simulink model "VB_RI_EKF_GNSS_INS25"  (R2023a)
settings: Solver=FixedStepAuto  StartTime=0  StopTime=200  FixedStep=0.01  RelTol=1e-3
InitFcn:
  | %resilient_initNavigation1216;
  | %init_param;
values from neighbouring files (symbols this model uses):
  C = zeros(n,m)    [utchol.m]
undefined symbols (not defined in the file or in its folder): dt, dtDelay, g0, gam0_rad, GNSSoutragetime, ISUS_flag, magnitude, p, P0, P0_RIEKF, param, pd0, pe0, phi0_rad, pn0, psi, psi0_rad, state_dim, vd0, ve0, vn0
libraries: simulink_extras x133, simulink x81, dspstat3 x81, sharedtransform x69, sharedTrackingLibrary x17, matrix_library x15, deeplib x6, dspfactors x4, aerolibconvert2 x4, aerolibtransform2 x4, dspsrcs4 x1
(part 7 of 32)

== system VB_RI_EKF_GNSS_INS25/ISUS_RIEKF3/INS propogation ==
  note: q(1:3)
  note: Data Split
  Sensor_data : Inport
  Measuemrnt Enable Flag : Inport  Port=2
  delta_state : Inport  Port=3
  Bus Creator : BusCreator  Inputs=7
  Bus Selector : BusSelector  OutputSignals=IMU_Data.gyro_B_rad/s_LPF,IMU_Data.accl_B_m/s2_LPF,MAGN_Data,QGC_sensor_reinit,GPS_Data.pos_N_gps,GPS_Data.pos_E_gps,GPS_Data.pos_D_gps,GPS_Data.vn_gps,GPS_Data.ve_gps,GPS_Data.vd_gps,VairspeedData,elevator_aileron_rudder_deg
  Bus Selector1 : BusSelector  OutputSignals=DCM_b_n
  Bus Selector2 : BusSelector  OutputSignals=delta_state.KFState_dtheta,delta_state.KFState_dv,delta_state.KFState_dp,delta_state.KFState_dg,delta_state.KFState_da
  Data Store Read2 : DataStoreRead  DataStoreName=GPS_enable_RIEKF  IndexOptions=Index vector (dialog)  Indices=1  OutputSizes=1
  Data Type Conversion : DataTypeConversion  OutDataTypeStr=single  SaturateOnIntegerOverflow=off  RndMeth=Floor
  Gain : Gain  Gain=0.1
  Gain1 : Gain  Gain=-1
  Gain2 : Gain  Gain=0.1
  Gain4 : Gain  Commented=on  Gain=-1
  Goto15 : Goto  Commented=on  GotoTag=dtheta
  Goto16 : Goto  Commented=on  GotoTag=dv
  Goto17 : Goto  Commented=on  GotoTag=dp
  Goto18 : Goto  Commented=on  GotoTag=dda
  Goto20 : Goto  Commented=on  GotoTag=ddg
  Init_PVQ : Subsystem
  Memory : Memory
  Mux : Mux  Inputs=3
  Mux1 : Mux  Inputs=3
  Reshape : Reshape  Commented=on
  Scope : Scope
  Selector : Selector  Commented=on  InputPortWidth=15  IndexOptions=Index vector (dialog)  Indices=[1 2 3]  OutputSizes=1
  Selector1 : Selector  Commented=on  InputPortWidth=15  IndexOptions=Index vector (dialog)  Indices=[4 5 6]  OutputSizes=1
  Selector2 : Selector  Commented=on  InputPortWidth=15  IndexOptions=Index vector (dialog)  Indices=[7 8 9]  OutputSizes=1
  Selector3 : Selector  Commented=on  InputPortWidth=15  IndexOptions=Index vector (dialog)  Indices=[10 11 12]  OutputSizes=1
  Selector4 : Selector  Commented=on  InputPortWidth=15  IndexOptions=Index vector (dialog)  Indices=[13 14 15]  OutputSizes=1
  accl bias compensation : Subsystem
  att update : Subsystem
  gyro bias compensation : Subsystem
  vel/pos update : Subsystem
  INSstate : Outport
  wires:
  delta_state/1 -> Memory/1
  Gain2/1 -> accl bias compensation/3(dda)
  Gain/1 -> gyro bias compensation/2(ddg)
  Gain4/1 -> Goto15/1
  Selector/1 -> Gain4/1
  Selector1/1 -> Goto16/1
  Selector2/1 -> Goto17/1
  Reshape/1 -> Selector2/1, Selector1/1, Selector3/1, Selector/1, Selector4/1
  Selector4/1 -> Goto18/1
  Selector3/1 -> Goto20/1
  Memory/1 -> Bus Selector2/1
  [dtheta] -> att update/1(dtheta)
  [dda] -> Gain2/1
  [ddg] -> Gain/1
  Bus Selector/12 -> [elevator_aileron_rudder_deg]  "<elevator_aileron_rudder_deg>"
  Bus Creator/1 -> INSstate/1
  Bus Selector/11 -> [TAS]  "<VairspeedData>"
  Gain1/1 -> [dtheta]
  [QGC_init] -> accl bias compensation/1(QGC_init), gyro bias compensation/4(QGC_init)
  [dtheta] -> vel/pos update/1(dtheta)
  Mux/1 -> [pos_NED]
  Init_PVQ/1(quat_0) -> att update/3(quat_0)
  [accl_raw] -> vel/pos update/3(Ab)
  [QGC_init] -> att update/4(init_flag)
  Bus Selector/10 -> Mux1/3  "<vd_gps>"
  [vel_NED] -> Data Type Conversion/1
  Bus Selector/7 -> Mux/3  "<pos_D_gps>"
  Bus Selector/8 -> Mux1/1  "<vn_gps>"
  Bus Selector/5 -> Mux/1  "<pos_N_gps>"
  [gyro_raw] -> att update/2(gyro)
  Bus Selector/6 -> Mux/2  "<pos_E_gps>"
  Bus Selector/3 -> [Magn]  "<MAGN_Data>"
  Mux1/1 -> [vel_NED]
  Sensor_data/1 -> Bus Selector/1
  [fbxyz] -> Init_PVQ/2(accl_B_m/s2_LPF)
  Init_PVQ/2(v0) -> vel/pos update/4(v0)
  Init_PVQ/3(p0) -> vel/pos update/5(p0)
  Bus Selector/9 -> Mux1/2  "<ve_gps>"
  [QGC_init] -> vel/pos update/6(QGC_init)
  [pos_NED] -> Init_PVQ/4(pos_NED)
  Data Type Conversion/1 -> Init_PVQ/5(vel_NED)
  [dp] -> vel/pos update/7(dp)
  [Magn] -> Init_PVQ/3(Magn_B_guess_LPF)
  Bus Selector/4 -> [QGC_init]  "<QGC_sensor_reinit>"
  Bus Selector/1 -> [gyro_raw]  "<gyro_B_rad/s_LPF>"
  Bus Selector1/1 -> vel/pos update/2(<DCM_b_n>)  "<DCM_b_n>"
  vel/pos update/2(V) -> Bus Creator/3  "INSstate_v"
  [dv] -> vel/pos update/8(dv)
  [QGC_init] -> Init_PVQ/1(QGC_sensor_reinit)
  vel/pos update/1(p_k) -> Bus Creator/2  "INSstste_p"
  [wxyz] -> Bus Creator/4  "INSstate_w"
  [fbxyz] -> Bus Creator/5  "INSstate_fb"
  att update/1(att_update1) -> Bus Selector1/1, Bus Creator/1  "RotationData"
  accl bias compensation/1(fb) -> [fbxyz]
  accl bias compensation/2(da) -> [da]
  Measuemrnt Enable Flag/1 -> gyro bias compensation/3(Measuemrnt Enable Flag)
  gyro bias compensation/1(wb) -> [wxyz]
  gyro bias compensation/2(dg) -> [dg]
  [dg] -> Bus Creator/6  "INSstate_dg"
  [da] -> Bus Creator/7  "INSstate_da"
  Bus Selector2/3 -> [dp], Scope/1  "<KFState_dp>"
  Bus Selector2/2 -> [dv]  "<KFState_dv>"
  Bus Selector2/1 -> Gain1/1  "<KFState_dtheta>"
  Bus Selector2/5 -> [dda]  "<KFState_da>"
  Bus Selector2/4 -> [ddg]  "<KFState_dg>"
  [gyro_raw] -> gyro bias compensation/1(raw <gyro_B_rad/s_LPF>)
  [accl_raw] -> accl bias compensation/2(raw <accl_B_m/s2_LPF>)
  Bus Selector/2 -> [accl_raw]  "<accl_B_m/s2_LPF>"

== system VB_RI_EKF_GNSS_INS25/ISUS_RIEKF3/INS propogation1 ==
  note: Data Split
  note: q(1:3)
  Sensor_data : Inport
  Measuemrnt Enable Flag : Inport  Port=2
  delta_state : Inport  Port=3
  Bus Creator : BusCreator  Inputs=7
  Bus Selector : BusSelector  OutputSignals=IMU_Data.gyro_B_rad/s_LPF,IMU_Data.accl_B_m/s2_LPF,MAGN_Data,QGC_sensor_reinit,GPS_Data.pos_N_gps,GPS_Data.pos_E_gps,GPS_Data.pos_D_gps,GPS_Data.vn_gps,GPS_Data.ve_gps,GPS_Data.vd_gps,VairspeedData,elevator_aileron_rudder_deg
  Bus Selector1 : BusSelector  OutputSignals=DCM_b_n
  Bus Selector2 : BusSelector  OutputSignals=delta_state.KFState_dtheta,delta_state.KFState_dv,delta_state.KFState_dp,delta_state.KFState_dg,delta_state.KFState_da
  Data Store Read2 : DataStoreRead  DataStoreName=GPS_enable_RIEKF  IndexOptions=Index vector (dialog)  Indices=1  OutputSizes=1
  Data Type Conversion : DataTypeConversion  OutDataTypeStr=single  SaturateOnIntegerOverflow=off  RndMeth=Floor
  Gain : Gain  Gain=0.1
  Gain1 : Gain  Gain=-1
  Gain2 : Gain  Gain=0.1
  Gain4 : Gain  Commented=on  Gain=-1
  Goto15 : Goto  Commented=on  GotoTag=dtheta
  Goto16 : Goto  Commented=on  GotoTag=dv
  Goto17 : Goto  Commented=on  GotoTag=dp
  Goto18 : Goto  Commented=on  GotoTag=dda
  Goto20 : Goto  Commented=on  GotoTag=ddg
  Init_PVQ : Subsystem
  Memory : Memory
  Mux : Mux  Inputs=3
  Mux1 : Mux  Inputs=3
  Reshape : Reshape  Commented=on
  Scope : Scope
  Selector : Selector  Commented=on  InputPortWidth=15  IndexOptions=Index vector (dialog)  Indices=[1 2 3]  OutputSizes=1
  Selector1 : Selector  Commented=on  InputPortWidth=15  IndexOptions=Index vector (dialog)  Indices=[4 5 6]  OutputSizes=1
  Selector2 : Selector  Commented=on  InputPortWidth=15  IndexOptions=Index vector (dialog)  Indices=[7 8 9]  OutputSizes=1
  Selector3 : Selector  Commented=on  InputPortWidth=15  IndexOptions=Index vector (dialog)  Indices=[10 11 12]  OutputSizes=1
  Selector4 : Selector  Commented=on  InputPortWidth=15  IndexOptions=Index vector (dialog)  Indices=[13 14 15]  OutputSizes=1
  accl bias compensation : Subsystem
  att update : Subsystem
  gyro bias compensation : Subsystem
  vel/pos update : Subsystem
  INSstate : Outport
  wires:
  Bus Selector/2 -> [accl_raw]  "<accl_B_m/s2_LPF>"
  [accl_raw] -> accl bias compensation/2(raw <accl_B_m/s2_LPF>)
  [gyro_raw] -> gyro bias compensation/1(raw <gyro_B_rad/s_LPF>)
  Bus Selector2/4 -> [ddg]  "<KFState_dg>"
  Bus Selector2/5 -> [dda]  "<KFState_da>"
  Bus Selector2/1 -> Gain1/1  "<KFState_dtheta>"
  Bus Selector2/2 -> [dv]  "<KFState_dv>"
  Bus Selector2/3 -> Scope/1, [dp]  "<KFState_dp>"
  [da] -> Bus Creator/7  "INSstate_da"
  [dg] -> Bus Creator/6  "INSstate_dg"
  gyro bias compensation/2(dg) -> [dg]
  gyro bias compensation/1(wb) -> [wxyz]
  Measuemrnt Enable Flag/1 -> gyro bias compensation/3(Measuemrnt Enable Flag)
  accl bias compensation/2(da) -> [da]
  accl bias compensation/1(fb) -> [fbxyz]
  att update/1(att_update1) -> Bus Creator/1, Bus Selector1/1  "RotationData"
  [fbxyz] -> Bus Creator/5  "INSstate_fb"
  [wxyz] -> Bus Creator/4  "INSstate_w"
  vel/pos update/1(p_k) -> Bus Creator/2  "INSstste_p"
  [QGC_init] -> Init_PVQ/1(QGC_sensor_reinit)
  [dv] -> vel/pos update/8(dv)
  vel/pos update/2(V) -> Bus Creator/3  "INSstate_v"
  Bus Selector1/1 -> vel/pos update/2(<DCM_b_n>)  "<DCM_b_n>"
  Bus Selector/1 -> [gyro_raw]  "<gyro_B_rad/s_LPF>"
  Bus Selector/4 -> [QGC_init]  "<QGC_sensor_reinit>"
  [Magn] -> Init_PVQ/3(Magn_B_guess_LPF)
  [dp] -> vel/pos update/7(dp)
  Data Type Conversion/1 -> Init_PVQ/5(vel_NED)
  [pos_NED] -> Init_PVQ/4(pos_NED)
  [QGC_init] -> vel/pos update/6(QGC_init)
  Bus Selector/9 -> Mux1/2  "<ve_gps>"
  Init_PVQ/3(p0) -> vel/pos update/5(p0)
  Init_PVQ/2(v0) -> vel/pos update/4(v0)
  [fbxyz] -> Init_PVQ/2(accl_B_m/s2_LPF)
  Sensor_data/1 -> Bus Selector/1
  Mux1/1 -> [vel_NED]
  Bus Selector/3 -> [Magn]  "<MAGN_Data>"
  Bus Selector/6 -> Mux/2  "<pos_E_gps>"
  [gyro_raw] -> att update/2(gyro)
  Bus Selector/5 -> Mux/1  "<pos_N_gps>"
  Bus Selector/8 -> Mux1/1  "<vn_gps>"
  Bus Selector/7 -> Mux/3  "<pos_D_gps>"
  [vel_NED] -> Data Type Conversion/1
  Bus Selector/10 -> Mux1/3  "<vd_gps>"
  [QGC_init] -> att update/4(init_flag)
  [accl_raw] -> vel/pos update/3(Ab)
  Init_PVQ/1(quat_0) -> att update/3(quat_0)
  Mux/1 -> [pos_NED]
  [dtheta] -> vel/pos update/1(dtheta)
  [QGC_init] -> gyro bias compensation/4(QGC_init), accl bias compensation/1(QGC_init)
  Gain1/1 -> [dtheta]
  Bus Selector/11 -> [TAS]  "<VairspeedData>"
  Bus Creator/1 -> INSstate/1
  Bus Selector/12 -> [elevator_aileron_rudder_deg]  "<elevator_aileron_rudder_deg>"
  [ddg] -> Gain/1
  [dda] -> Gain2/1
  [dtheta] -> att update/1(dtheta)
  Memory/1 -> Bus Selector2/1
  Selector3/1 -> Goto20/1
  Selector4/1 -> Goto18/1
  Reshape/1 -> Selector4/1, Selector/1, Selector3/1, Selector1/1, Selector2/1
  Selector2/1 -> Goto17/1
  Selector1/1 -> Goto16/1
  Selector/1 -> Gain4/1
  Gain4/1 -> Goto15/1
  Gain/1 -> gyro bias compensation/2(ddg)
  Gain2/1 -> accl bias compensation/3(dda)
  delta_state/1 -> Memory/1

== system VB_RI_EKF_GNSS_INS25/ISUS_RIEKF3/INS propogation2 ==
  note: q(1:3)
  note: Data Split
  Sensor_data : Inport
  Measuemrnt Enable Flag : Inport  Port=2
  delta_state : Inport  Port=3
  Bus Creator : BusCreator  Inputs=7
  Bus Selector : BusSelector  OutputSignals=IMU_Data.gyro_B_rad/s_LPF,IMU_Data.accl_B_m/s2_LPF,MAGN_Data,QGC_sensor_reinit,GPS_Data.pos_N_gps,GPS_Data.pos_E_gps,GPS_Data.pos_D_gps,GPS_Data.vn_gps,GPS_Data.ve_gps,GPS_Data.vd_gps,VairspeedData,elevator_aileron_rudder_deg
  Bus Selector1 : BusSelector  OutputSignals=DCM_b_n
  Bus Selector2 : BusSelector  OutputSignals=delta_state.KFState_dtheta,delta_state.KFState_dv,delta_state.KFState_dp,delta_state.KFState_dg,delta_state.KFState_da
  Data Store Read2 : DataStoreRead  DataStoreName=GPS_enable_RIEKF  IndexOptions=Index vector (dialog)  Indices=1  OutputSizes=1
  Data Type Conversion : DataTypeConversion  OutDataTypeStr=single  SaturateOnIntegerOverflow=off  RndMeth=Floor
  Gain : Gain  Gain=0.1
  Gain1 : Gain  Gain=-1
  Gain2 : Gain  Gain=0.1
  Gain4 : Gain  Commented=on  Gain=-1
  Goto15 : Goto  Commented=on  GotoTag=dtheta
  Goto16 : Goto  Commented=on  GotoTag=dv
  Goto17 : Goto  Commented=on  GotoTag=dp
  Goto18 : Goto  Commented=on  GotoTag=dda
  Goto20 : Goto  Commented=on  GotoTag=ddg
  Init_PVQ : Subsystem
  Memory : Memory
  Mux : Mux  Inputs=3
  Mux1 : Mux  Inputs=3
  Reshape : Reshape  Commented=on
  Scope : Scope
  Selector : Selector  Commented=on  InputPortWidth=15  IndexOptions=Index vector (dialog)  Indices=[1 2 3]  OutputSizes=1
  Selector1 : Selector  Commented=on  InputPortWidth=15  IndexOptions=Index vector (dialog)  Indices=[4 5 6]  OutputSizes=1
  Selector2 : Selector  Commented=on  InputPortWidth=15  IndexOptions=Index vector (dialog)  Indices=[7 8 9]  OutputSizes=1
  Selector3 : Selector  Commented=on  InputPortWidth=15  IndexOptions=Index vector (dialog)  Indices=[10 11 12]  OutputSizes=1
  Selector4 : Selector  Commented=on  InputPortWidth=15  IndexOptions=Index vector (dialog)  Indices=[13 14 15]  OutputSizes=1
  accl bias compensation : Subsystem
  att update : Subsystem
  gyro bias compensation : Subsystem
  vel/pos update : Subsystem
  INSstate : Outport
  wires:
  delta_state/1 -> Memory/1
  Gain2/1 -> accl bias compensation/3(dda)
  Gain/1 -> gyro bias compensation/2(ddg)
  Gain4/1 -> Goto15/1
  Selector/1 -> Gain4/1
  Selector1/1 -> Goto16/1
  Selector2/1 -> Goto17/1
  Reshape/1 -> Selector2/1, Selector1/1, Selector3/1, Selector/1, Selector4/1
  Selector4/1 -> Goto18/1
  Selector3/1 -> Goto20/1
  Memory/1 -> Bus Selector2/1
  [dtheta] -> att update/1(dtheta)
  [dda] -> Gain2/1
  [ddg] -> Gain/1
  Bus Selector/12 -> [elevator_aileron_rudder_deg]  "<elevator_aileron_rudder_deg>"
  Bus Creator/1 -> INSstate/1
  Bus Selector/11 -> [TAS]  "<VairspeedData>"
  Gain1/1 -> [dtheta]
  [QGC_init] -> accl bias compensation/1(QGC_init), gyro bias compensation/4(QGC_init)
  [dtheta] -> vel/pos update/1(dtheta)
  Mux/1 -> [pos_NED]
  Init_PVQ/1(quat_0) -> att update/3(quat_0)
  [accl_raw] -> vel/pos update/3(Ab)
  [QGC_init] -> att update/4(init_flag)
  Bus Selector/10 -> Mux1/3  "<vd_gps>"
  [vel_NED] -> Data Type Conversion/1
  Bus Selector/7 -> Mux/3  "<pos_D_gps>"
  Bus Selector/8 -> Mux1/1  "<vn_gps>"
  Bus Selector/5 -> Mux/1  "<pos_N_gps>"
  [gyro_raw] -> att update/2(gyro)
  Bus Selector/6 -> Mux/2  "<pos_E_gps>"
  Bus Selector/3 -> [Magn]  "<MAGN_Data>"
  Mux1/1 -> [vel_NED]
  Sensor_data/1 -> Bus Selector/1
  [fbxyz] -> Init_PVQ/2(accl_B_m/s2_LPF)
  Init_PVQ/2(v0) -> vel/pos update/4(v0)
  Init_PVQ/3(p0) -> vel/pos update/5(p0)
  Bus Selector/9 -> Mux1/2  "<ve_gps>"
  [QGC_init] -> vel/pos update/6(QGC_init)
  [pos_NED] -> Init_PVQ/4(pos_NED)
  Data Type Conversion/1 -> Init_PVQ/5(vel_NED)
  [dp] -> vel/pos update/7(dp)
  [Magn] -> Init_PVQ/3(Magn_B_guess_LPF)
  Bus Selector/4 -> [QGC_init]  "<QGC_sensor_reinit>"
  Bus Selector/1 -> [gyro_raw]  "<gyro_B_rad/s_LPF>"
  Bus Selector1/1 -> vel/pos update/2(<DCM_b_n>)  "<DCM_b_n>"
  vel/pos update/2(V) -> Bus Creator/3  "INSstate_v"
  [dv] -> vel/pos update/8(dv)
  [QGC_init] -> Init_PVQ/1(QGC_sensor_reinit)
  vel/pos update/1(p_k) -> Bus Creator/2  "INSstste_p"
  [wxyz] -> Bus Creator/4  "INSstate_w"
  [fbxyz] -> Bus Creator/5  "INSstate_fb"
  att update/1(att_update1) -> Bus Selector1/1, Bus Creator/1  "RotationData"
  accl bias compensation/1(fb) -> [fbxyz]
  accl bias compensation/2(da) -> [da]
  Measuemrnt Enable Flag/1 -> gyro bias compensation/3(Measuemrnt Enable Flag)
  gyro bias compensation/1(wb) -> [wxyz]
  gyro bias compensation/2(dg) -> [dg]
  [dg] -> Bus Creator/6  "INSstate_dg"
  [da] -> Bus Creator/7  "INSstate_da"
  Bus Selector2/3 -> [dp], Scope/1  "<KFState_dp>"
  Bus Selector2/2 -> [dv]  "<KFState_dv>"
  Bus Selector2/1 -> Gain1/1  "<KFState_dtheta>"
  Bus Selector2/5 -> [dda]  "<KFState_da>"
  Bus Selector2/4 -> [ddg]  "<KFState_dg>"
  [gyro_raw] -> gyro bias compensation/1(raw <gyro_B_rad/s_LPF>)
  [accl_raw] -> accl bias compensation/2(raw <accl_B_m/s2_LPF>)
  Bus Selector/2 -> [accl_raw]  "<accl_B_m/s2_LPF>"

== system VB_RI_EKF_GNSS_INS25/ISUS_RIEKF3/INS propogation3 ==
  note: Data Split
  note: q(1:3)
  Sensor_data : Inport
  Measuemrnt Enable Flag : Inport  Port=2
  delta_state : Inport  Port=3
  Bus Creator : BusCreator  Inputs=7
  Bus Selector : BusSelector  OutputSignals=IMU_Data.gyro_B_rad/s_LPF,IMU_Data.accl_B_m/s2_LPF,MAGN_Data,QGC_sensor_reinit,GPS_Data.pos_N_gps,GPS_Data.pos_E_gps,GPS_Data.pos_D_gps,GPS_Data.vn_gps,GPS_Data.ve_gps,GPS_Data.vd_gps,VairspeedData,elevator_aileron_rudder_deg
  Bus Selector1 : BusSelector  OutputSignals=DCM_b_n
  Bus Selector2 : BusSelector  OutputSignals=delta_state.KFState_dtheta,delta_state.KFState_dv,delta_state.KFState_dp,delta_state.KFState_dg,delta_state.KFState_da
  Data Store Read2 : DataStoreRead  DataStoreName=GPS_enable_RIEKF  IndexOptions=Index vector (dialog)  Indices=1  OutputSizes=1
  Data Type Conversion : DataTypeConversion  OutDataTypeStr=single  SaturateOnIntegerOverflow=off  RndMeth=Floor
  Gain : Gain  Gain=0.1
  Gain1 : Gain  Gain=-1
  Gain2 : Gain  Gain=0.1
  Gain4 : Gain  Commented=on  Gain=-1
  Goto15 : Goto  Commented=on  GotoTag=dtheta
  Goto16 : Goto  Commented=on  GotoTag=dv
  Goto17 : Goto  Commented=on  GotoTag=dp
  Goto18 : Goto  Commented=on  GotoTag=dda
  Goto20 : Goto  Commented=on  GotoTag=ddg
  Init_PVQ : Subsystem
  Memory : Memory
  Mux : Mux  Inputs=3
  Mux1 : Mux  Inputs=3
  Reshape : Reshape  Commented=on
  Scope : Scope
  Selector : Selector  Commented=on  InputPortWidth=15  IndexOptions=Index vector (dialog)  Indices=[1 2 3]  OutputSizes=1
  Selector1 : Selector  Commented=on  InputPortWidth=15  IndexOptions=Index vector (dialog)  Indices=[4 5 6]  OutputSizes=1
  Selector2 : Selector  Commented=on  InputPortWidth=15  IndexOptions=Index vector (dialog)  Indices=[7 8 9]  OutputSizes=1
  Selector3 : Selector  Commented=on  InputPortWidth=15  IndexOptions=Index vector (dialog)  Indices=[10 11 12]  OutputSizes=1
  Selector4 : Selector  Commented=on  InputPortWidth=15  IndexOptions=Index vector (dialog)  Indices=[13 14 15]  OutputSizes=1
  accl bias compensation : Subsystem
  att update : Subsystem
  gyro bias compensation : Subsystem
  vel/pos update : Subsystem
  INSstate : Outport
  wires:
  Bus Selector/2 -> [accl_raw]  "<accl_B_m/s2_LPF>"
  [accl_raw] -> accl bias compensation/2(raw <accl_B_m/s2_LPF>)
  [gyro_raw] -> gyro bias compensation/1(raw <gyro_B_rad/s_LPF>)
  Bus Selector2/4 -> [ddg]  "<KFState_dg>"
  Bus Selector2/5 -> [dda]  "<KFState_da>"
  Bus Selector2/1 -> Gain1/1  "<KFState_dtheta>"
  Bus Selector2/2 -> [dv]  "<KFState_dv>"
  Bus Selector2/3 -> Scope/1, [dp]  "<KFState_dp>"
  [da] -> Bus Creator/7  "INSstate_da"
  [dg] -> Bus Creator/6  "INSstate_dg"
  gyro bias compensation/2(dg) -> [dg]
  gyro bias compensation/1(wb) -> [wxyz]
  Measuemrnt Enable Flag/1 -> gyro bias compensation/3(Measuemrnt Enable Flag)
  accl bias compensation/2(da) -> [da]
  accl bias compensation/1(fb) -> [fbxyz]
  att update/1(att_update1) -> Bus Creator/1, Bus Selector1/1  "RotationData"
  [fbxyz] -> Bus Creator/5  "INSstate_fb"
  [wxyz] -> Bus Creator/4  "INSstate_w"
  vel/pos update/1(p_k) -> Bus Creator/2  "INSstste_p"
  [QGC_init] -> Init_PVQ/1(QGC_sensor_reinit)
  [dv] -> vel/pos update/8(dv)
  vel/pos update/2(V) -> Bus Creator/3  "INSstate_v"
  Bus Selector1/1 -> vel/pos update/2(<DCM_b_n>)  "<DCM_b_n>"
  Bus Selector/1 -> [gyro_raw]  "<gyro_B_rad/s_LPF>"
  Bus Selector/4 -> [QGC_init]  "<QGC_sensor_reinit>"
  [Magn] -> Init_PVQ/3(Magn_B_guess_LPF)
  [dp] -> vel/pos update/7(dp)
  Data Type Conversion/1 -> Init_PVQ/5(vel_NED)
  [pos_NED] -> Init_PVQ/4(pos_NED)
  [QGC_init] -> vel/pos update/6(QGC_init)
  Bus Selector/9 -> Mux1/2  "<ve_gps>"
  Init_PVQ/3(p0) -> vel/pos update/5(p0)
  Init_PVQ/2(v0) -> vel/pos update/4(v0)
  [fbxyz] -> Init_PVQ/2(accl_B_m/s2_LPF)
  Sensor_data/1 -> Bus Selector/1
  Mux1/1 -> [vel_NED]
  Bus Selector/3 -> [Magn]  "<MAGN_Data>"
  Bus Selector/6 -> Mux/2  "<pos_E_gps>"
  [gyro_raw] -> att update/2(gyro)
  Bus Selector/5 -> Mux/1  "<pos_N_gps>"
  Bus Selector/8 -> Mux1/1  "<vn_gps>"
  Bus Selector/7 -> Mux/3  "<pos_D_gps>"
  [vel_NED] -> Data Type Conversion/1
  Bus Selector/10 -> Mux1/3  "<vd_gps>"
  [QGC_init] -> att update/4(init_flag)
  [accl_raw] -> vel/pos update/3(Ab)
  Init_PVQ/1(quat_0) -> att update/3(quat_0)
  Mux/1 -> [pos_NED]
  [dtheta] -> vel/pos update/1(dtheta)
  [QGC_init] -> gyro bias compensation/4(QGC_init), accl bias compensation/1(QGC_init)
  Gain1/1 -> [dtheta]
  Bus Selector/11 -> [TAS]  "<VairspeedData>"
  Bus Creator/1 -> INSstate/1
  Bus Selector/12 -> [elevator_aileron_rudder_deg]  "<elevator_aileron_rudder_deg>"
  [ddg] -> Gain/1
  [dda] -> Gain2/1
  [dtheta] -> att update/1(dtheta)
  Memory/1 -> Bus Selector2/1
  Selector3/1 -> Goto20/1
  Selector4/1 -> Goto18/1
  Reshape/1 -> Selector4/1, Selector/1, Selector3/1, Selector1/1, Selector2/1
  Selector2/1 -> Goto17/1
  Selector1/1 -> Goto16/1
  Selector/1 -> Gain4/1
  Gain4/1 -> Goto15/1
  Gain/1 -> gyro bias compensation/2(ddg)
  Gain2/1 -> accl bias compensation/3(dda)
  delta_state/1 -> Memory/1

== system VB_RI_EKF_GNSS_INS25/ISUS_RIEKF3/Subsystem ==
  EKFstate_M1 : Inport
  EKFstate_M2 : Inport  Port=2
  EKFstate_M3 : Inport  Port=3
  Bus Selector : BusSelector  OutputSignals=delta_state,covariance,beta1
  Bus Selector1 : BusSelector  OutputSignals=delta_state,covariance,m_innov_z0,Sk_z0,beta2
  Bus Selector2 : BusSelector  OutputSignals=delta_state,covariance,m_innov_z0,Sk_z0,beta3
  Constant1 : Constant  Value=P0_RIEKF  OutDataTypeStr=single
  Constant6 : Constant  Value=zeros(15,1)  OutDataTypeStr=single
  Constant7 : Constant  Value=P0_RIEKF  OutDataTypeStr=single
  Delay{,1..3,5..7} (7 alike) : Delay  DelayLength=1  InitialConditionSource=Input port
      settings: InputPortMap=u0,p4
  Display : Display
  Display1 : Display
  Display2 : Display
  Gain : Gain  Gain=3
  ISIU : Subsystem
  Reshape2 : Reshape  OutputDimensionality=Column vector (2-D)
  Subsystem : Subsystem
  Subsystem1 : Subsystem
  Subsystem2 : Subsystem
  Subsystem3 : Subsystem
  P_mixed_RIEKF_M1 : Outport
  X_mixed_RIEKF_M1 : Outport  Port=2
  P_mixed_RIEKF_M2 : Outport  Port=3
  X_mixed_RIEKF_M2 : Outport  Port=4
  xk_k : Outport  Port=5
  pk_k : Outport  Port=6
  X_mixed_RIEKF_M3 : Outport  Port=7
  P_mixed_RIEKF_M3 : Outport  Port=8
  beta_1 : Outport  Port=9
  beta_2 : Outport  Port=10
  beta_3 : Outport  Port=11
  wires:
  Bus Selector2/1 -> ISIU/3(xk_k_3)  "<delta_state>"
  EKFstate_M3/1 -> Bus Selector2/1
  ISIU/8(pk_k_o3) -> Delay7/1
  Delay7/1 -> P_mixed_RIEKF_M3/1
  ISIU/5(xk_k_o3) -> Delay6/1
  Reshape2/1 -> Delay/2, Delay3/2, Delay6/2
  Delay6/1 -> Subsystem3/1(X_mixed_RIEKF_M1)
  ISIU/1(xk_k) -> Subsystem/1(X_mixed_RIEKF_M1)
  Subsystem/1(Out1) -> xk_k/1  "xk_k"
  Constant1/1 -> Delay5/2
  ISIU/2(pk_k) -> Delay5/1
  Delay5/1 -> pk_k/1
  Delay3/1 -> Subsystem2/1(X_mixed_RIEKF_M1)
  Delay1/1 -> P_mixed_RIEKF_M1/1
  ISIU/3(xk_k_o1) -> Delay/1  "X_mixed_RIEKF_M1"
  EKFstate_M1/1 -> Bus Selector/1
  ISIU/6(pk_k_o1) -> Delay1/1
  Bus Selector/1 -> ISIU/1(xk_k_1)  "<delta_state>"
  Delay2/1 -> P_mixed_RIEKF_M2/1
  Constant6/1 -> Reshape2/1
  ISIU/7(pk_k_o2) -> Delay2/1
  ISIU/4(xk_k_o2) -> Delay3/1  "X_mixed_RIEKF_M2"
  EKFstate_M2/1 -> Bus Selector1/1
  Delay/1 -> Subsystem1/1(X_mixed_RIEKF_M1)
  Bus Selector1/1 -> ISIU/2(xk_k_2)  "<delta_state>"
  Constant7/1 -> Gain/1
  Bus Selector/2 -> ISIU/4(pk_k_1)  "<covariance>"
  Bus Selector1/2 -> ISIU/5(pk_k_2)  "<covariance>"
  Bus Selector2/2 -> ISIU/6(pk_k_3)  "<covariance>"
  Subsystem1/1(Out1) -> X_mixed_RIEKF_M1/1  "xk_k"
  Subsystem2/1(Out1) -> X_mixed_RIEKF_M2/1  "xk_k"
  Subsystem3/1(Out1) -> X_mixed_RIEKF_M3/1  "xk_k"
  Gain/1 -> Delay1/2, Delay2/2, Delay7/2
  Bus Selector/3 -> ISIU/7(beta1)  "<beta1>"
  Bus Selector1/5 -> ISIU/8(beta2)  "<beta2>"
  Bus Selector2/5 -> ISIU/9(beta3)  "<beta3>"
  ISIU/9(beta_1) -> Display/1, beta_1/1
  ISIU/10(beta_2) -> Display1/1, beta_2/1
  ISIU/11(beta_3) -> Display2/1, beta_3/1

== system VB_RI_EKF_GNSS_INS25/No.1_Sensor_Data_Process/GPS_Data_Process ==
  note: GPS_fixtype:
      | 0: 定位不可用或无效
      | 1:单点定位
      | 2:伪距差分
      | 4:RTK固定解
  GPS_Vecef_m/s : Inport
  GPS_LLA_rad : Inport  Port=2
  GPS_fixtype : Inport  Port=3
  hdop_GPS : Inport  Port=4
  QGC_sensor_reinit : Inport  Port=5
  Bus Creator : BusCreator  Inputs=13
  Demux : Demux  Outputs=3
  Demux1 : Demux  Outputs=3
  Demux3 : Demux  Outputs=3
  GPS_fixtype1 : InportShadow  Port=3
  LLA2NED : Subsystem
  heading_GPS : Subsystem
  GPS_Data : Outport
  GPS0 : Outport  Port=2
  GPS_noerr : Outport  Port=3
  wires:
  hdop_GPS/1 -> Bus Creator/13  "hdop_GPS"
  heading_GPS/2(heading_GPS_valid) -> Bus Creator/11  "heading_GPS_valid"
  heading_GPS/1(heading_GPS_rad) -> Bus Creator/10  "heading_GPS_rad"
  LLA2NED/2(gpsvNEDout) -> heading_GPS/1(Vned), Demux/1
  GPS_Vecef_m/s/1 -> LLA2NED/3(GPS_Vecef_m/s)
  Demux1/3 -> Bus Creator/6  "pos_D_gps"
  Demux1/2 -> Bus Creator/5  "pos_E_gps"
  Demux1/1 -> Bus Creator/4  "pos_N_gps"
  QGC_sensor_reinit/1 -> LLA2NED/4(QGC_sensor_reinit)  "QGC_sensor_reinit"
  GPS_fixtype/1 -> Bus Creator/12  "fixtype_gps"
  Demux3/1 -> Bus Creator/1  "lat_gps"
  Demux3/2 -> Bus Creator/2  "lon_gps"
  Demux/2 -> Bus Creator/8  "ve_gps"
  GPS_LLA_rad/1 -> LLA2NED/1(gps_LLA_rad), Demux3/1
  Demux/1 -> Bus Creator/7  "vn_gps"
  Demux/3 -> Bus Creator/9  "vd_gps"
  Demux3/3 -> Bus Creator/3  "H_gps"
  Bus Creator/1 -> GPS_Data/1
  GPS_fixtype1/1 -> LLA2NED/2(GPSfixtype)  "fixtype_gps"
  LLA2NED/1("gpsposNEDout ") -> Demux1/1
  LLA2NED/3(GPS0) -> GPS0/1
  LLA2NED/4(gpsposNED_noerr) -> GPS_noerr/1

== system VB_RI_EKF_GNSS_INS25/No.1_Sensor_Data_Process/IMU_Data_Process ==
  gyro_B_rad/s_ori : Inport
  accl_B_m/s_ori : Inport  Port=2
  Bias Eliminate : Subsystem
  Bus Creator : BusCreator  Inputs=2
  accl_preprocessing2 : Subsystem  Commented=on
  gyro_preprocessing2 : Subsystem  Commented=on
  IMU_Data : Outport  PortDimensions=6
  wires:
  gyro_B_rad/s_ori/1 -> Bias Eliminate/1(gyro_B_rad/s_ori)  "gyro_B_rad/s_LPF"
  Bias Eliminate/1(Out1) -> Bus Creator/1  "gyro_B_rad/s_LPF"
  accl_B_m/s_ori/1 -> Bus Creator/2  "accl_B_m/s2_LPF"
  Bus Creator/1 -> IMU_Data/1

== system VB_RI_EKF_GNSS_INS25/No.1_Sensor_Data_Process/Magn_Data_Process ==
  magn_B_guass_ori : Inport
  Data Type Conversion : DataTypeConversion  OutDataTypeStr=single  SaturateOnIntegerOverflow=off  RndMeth=Floor
  MATLAB Function1 : MATLAB Function  Commented=on  TreatAsAtomicUnit=on
  Magn_preprocessing : Subsystem
  MAGN_Data : Outport
  wires:
  magn_B_guass_ori/1 -> Data Type Conversion/1, Magn_preprocessing/1(Magn_B_rad/s_ori)
  Data Type Conversion/1 -> MAGN_Data/1

== system VB_RI_EKF_GNSS_INS25/No.1_Sensor_Data_Process/Subsystem ==
  Vairspeed : Inport
  Constant : Constant  Value=0  OutDataTypeStr=single
  Mux : Mux  Inputs=3
  TD_baro : Subsystem
  Terminator : Terminator
  VairspeedData : Outport
  wires:
  TD_baro/2(H_baro_TD) -> Mux/1
  Constant/1 -> Mux/3, Mux/2
  Mux/1 -> VairspeedData/1  "VairspeedData"
  Vairspeed/1 -> TD_baro/1(H_baro)
  TD_baro/1(vH_baro_TD) -> Terminator/1  "vH_baro_m/s_TD"

== system VB_RI_EKF_GNSS_INS25/No.1_Sensor_Data_Process/TOF_Data_Process ==
  TOF_mm_ori : Inport
  QGC_sensor_reinit : Inport  Port=2
  Bus Creator1 : BusCreator  Inputs=4
  Data Type Conversion : DataTypeConversion  OutDataTypeStr=uint8  SaturateOnIntegerOverflow=off  RndMeth=Floor
  Data Type Conversion1 : DataTypeConversion  OutDataTypeStr=single  SaturateOnIntegerOverflow=off  RndMeth=Floor
  Demux : Demux  Outputs=3
  Gain : Gain  Gain=0.01
  Scope : Scope  NumInputPorts=2
  Scope1 : Scope  NumInputPorts=2
  Sum : Sum  Inputs=|-+
  TD_baro : Subsystem
  reinit_TOF : Subsystem
  TOF_Data : Outport
  wires:
  Sum/1 -> Data Type Conversion1/1, Scope1/2  "TOF_Dist_m"
  reinit_TOF/1(dataout) -> Sum/1, Scope1/1
  QGC_sensor_reinit/1 -> reinit_TOF/1(QGC_sensor_reinit)
  Data Type Conversion/1 -> Bus Creator1/4  "TOF_sts"
  Gain/1 -> reinit_TOF/2(Data), Sum/2  "TOF_Dist_m"
  TD_baro/1(vH_TOF_TD) -> Bus Creator1/1, Scope/1  "vH_TOF_m/s_TD"
  Bus Creator1/1 -> TOF_Data/1  "TOF_Data"
  Demux/2 -> Bus Creator1/3  "TOF_Inten"
  TOF_mm_ori/1 -> Demux/1
  Demux/1 -> Gain/1
  Demux/3 -> Data Type Conversion/1  "TOF_sts"
  TD_baro/2(H_TOF_TD) -> Scope/2, Bus Creator1/2  "H_TOF_TD"
  Data Type Conversion1/1 -> TD_baro/1(H_TOF)  "补偿姿态前"

== system VB_RI_EKF_GNSS_INS25/No.1_Sensor_Data_Process/baro_Data_Process ==
  baro : Inport
  QGC_sensor_reinit : Inport  Port=2
  baro_tem : Inport  Port=3
  Bus Creator : BusCreator  Inputs=2
  Constant : Constant  Value=0  OutDataTypeStr=single
  From Workspace : FromWorkspace  Commented=on  VariableName=[All.t',All.Alt_Ps]
  Gain : Gain  Gain=0.01
  Pressure2Height : Subsystem
  Scope : Scope
  Scope1 : Scope  Commented=on  NumInputPorts=2
  Sum : Sum  Inputs=|+-
  Sum1 : Sum  Commented=on  Inputs=|+-
  Sum2 : Sum  Inputs=|+-
  Switch : Switch  Criteria=u2 > Threshold  Threshold=31  SaturateOnIntegerOverflow=off  InputSameDT=off
  TD_baro : Subsystem
  TemCompensate1 : Subsystem
  reinit_baro0 : Subsystem
  reinit_baro1 : Subsystem  Commented=on
  BARO_Data : Outport  PortDimensions=2
  wires:
  baro_tem/1 -> TemCompensate1/1(baro_tem), Switch/2  "AFCbarotem"
  Pressure2Height/1(H_baro) -> TD_baro/1(H_baro)  "AFC4"
  Switch/1 -> Sum2/2
  baro/1 -> Gain/1  "AFC4"
  Constant/1 -> Switch/1
  TemCompensate1/1(bias) -> Switch/3
  Sum2/1 -> Sum/1, reinit_baro0/2(Data)
  TD_baro/2(H_baro_TD) -> Sum2/1  "H_baro_TD"
  Sum/1 -> Scope1/2, Scope/1, Bus Creator/2  "H_baro_TD"
  reinit_baro0/1(dataout) -> Sum/2
  QGC_sensor_reinit/1 -> reinit_baro1/1(QGC_sensor_reinit), reinit_baro0/1(QGC_sensor_reinit)
  Bus Creator/1 -> BARO_Data/1
  Gain/1 -> Pressure2Height/1(baro)
  TD_baro/1(vH_baro_TD) -> Bus Creator/1  "vH_baro_m/s_TD"
  From Workspace/1 -> reinit_baro1/2(Data), Sum1/1
  reinit_baro1/1(dataout) -> Sum1/2
  Sum1/1 -> Scope1/1

== system VB_RI_EKF_GNSS_INS25/No.1_Sensor_Data_Process1/GPS_Data_Process ==
  note: GPS_fixtype:
      | 0: 定位不可用或无效
      | 1:单点定位
      | 2:伪距差分
      | 4:RTK固定解
  GPS_Vecef_m/s : Inport
  GPS_LLA_rad : Inport  Port=2
  GPS_fixtype : Inport  Port=3
  hdop_GPS : Inport  Port=4
  QGC_sensor_reinit : Inport  Port=5
  GPS0 : Inport  Port=6
  Bus Creator : BusCreator  Inputs=13
  Demux : Demux  Outputs=3
  Demux1 : Demux  Outputs=3
  Demux3 : Demux  Outputs=3
  GPS_fixtype1 : InportShadow  Port=3
  LLA2NED : Subsystem
  heading_GPS : Subsystem
  GPS_Data : Outport
  wires:
  LLA2NED/1("gpsposNEDout ") -> Demux1/1
  GPS_fixtype1/1 -> LLA2NED/2(GPSfixtype)  "fixtype_gps"
  Bus Creator/1 -> GPS_Data/1
  Demux3/3 -> Bus Creator/3  "H_gps"
  Demux/3 -> Bus Creator/9  "vd_gps"
  Demux/1 -> Bus Creator/7  "vn_gps"
  GPS_LLA_rad/1 -> Demux3/1, LLA2NED/1(gps_LLA_rad)
  Demux/2 -> Bus Creator/8  "ve_gps"
  Demux3/2 -> Bus Creator/2  "lon_gps"
  Demux3/1 -> Bus Creator/1  "lat_gps"
  GPS_fixtype/1 -> Bus Creator/12  "fixtype_gps"
  QGC_sensor_reinit/1 -> LLA2NED/4(QGC_sensor_reinit)  "QGC_sensor_reinit"
  Demux1/1 -> Bus Creator/4  "pos_N_gps"
  Demux1/2 -> Bus Creator/5  "pos_E_gps"
  Demux1/3 -> Bus Creator/6  "pos_D_gps"
  GPS_Vecef_m/s/1 -> LLA2NED/3(GPS_Vecef_m/s)
  LLA2NED/2(gpsvNEDout) -> Demux/1, heading_GPS/1(Vned)
  heading_GPS/1(heading_GPS_rad) -> Bus Creator/10  "heading_GPS_rad"
  heading_GPS/2(heading_GPS_valid) -> Bus Creator/11  "heading_GPS_valid"
  hdop_GPS/1 -> Bus Creator/13  "hdop_GPS"
  GPS0/1 -> LLA2NED/5(GPS0)

== system VB_RI_EKF_GNSS_INS25/No.1_Sensor_Data_Process1/IMU_Data_Process ==
  gyro_B_rad/s_ori : Inport
  accl_B_m/s_ori : Inport  Port=2
  Bias Eliminate : Subsystem
  Bus Creator : BusCreator  Inputs=2
  accl_preprocessing2 : Subsystem  Commented=on
  gyro_preprocessing2 : Subsystem  Commented=on
  IMU_Data : Outport  PortDimensions=6
  wires:
  Bus Creator/1 -> IMU_Data/1
  accl_B_m/s_ori/1 -> Bus Creator/2  "accl_B_m/s2_LPF"
  Bias Eliminate/1(Out1) -> Bus Creator/1  "gyro_B_rad/s_LPF"
  gyro_B_rad/s_ori/1 -> Bias Eliminate/1(gyro_B_rad/s_ori)  "gyro_B_rad/s_LPF"

== system VB_RI_EKF_GNSS_INS25/No.1_Sensor_Data_Process1/Magn_Data_Process ==
  magn_B_guass_ori : Inport
  Data Type Conversion : DataTypeConversion  OutDataTypeStr=single  SaturateOnIntegerOverflow=off  RndMeth=Floor
  MATLAB Function1 : MATLAB Function  Commented=on  TreatAsAtomicUnit=on
  Magn_preprocessing : Subsystem
  MAGN_Data : Outport
  wires:
  Data Type Conversion/1 -> MAGN_Data/1
  magn_B_guass_ori/1 -> Magn_preprocessing/1(Magn_B_rad/s_ori), Data Type Conversion/1

== system VB_RI_EKF_GNSS_INS25/No.1_Sensor_Data_Process1/Subsystem ==
  Vairspeed : Inport
  Constant : Constant  Value=0  OutDataTypeStr=single
  Mux : Mux  Inputs=3
  TD_baro : Subsystem
  Terminator : Terminator
  VairspeedData : Outport
  wires:
  TD_baro/1(vH_baro_TD) -> Terminator/1  "vH_baro_m/s_TD"
  Vairspeed/1 -> TD_baro/1(H_baro)
  Mux/1 -> VairspeedData/1  "VairspeedData"
  Constant/1 -> Mux/2, Mux/3
  TD_baro/2(H_baro_TD) -> Mux/1

== system VB_RI_EKF_GNSS_INS25/No.1_Sensor_Data_Process1/TOF_Data_Process ==
  TOF_mm_ori : Inport
  QGC_sensor_reinit : Inport  Port=2
  Bus Creator1 : BusCreator  Inputs=4
  Data Type Conversion : DataTypeConversion  OutDataTypeStr=uint8  SaturateOnIntegerOverflow=off  RndMeth=Floor
  Data Type Conversion1 : DataTypeConversion  OutDataTypeStr=single  SaturateOnIntegerOverflow=off  RndMeth=Floor
  Demux : Demux  Outputs=3
  Gain : Gain  Gain=0.01
  Scope : Scope  NumInputPorts=2
  Scope1 : Scope  NumInputPorts=2
  Sum : Sum  Inputs=|-+
  TD_baro : Subsystem
  reinit_TOF : Subsystem
  TOF_Data : Outport
  wires:
  Data Type Conversion1/1 -> TD_baro/1(H_TOF)  "补偿姿态前"
  TD_baro/2(H_TOF_TD) -> Bus Creator1/2, Scope/2  "H_TOF_TD"
  Demux/3 -> Data Type Conversion/1  "TOF_sts"
  Demux/1 -> Gain/1
  TOF_mm_ori/1 -> Demux/1
  Demux/2 -> Bus Creator1/3  "TOF_Inten"
  Bus Creator1/1 -> TOF_Data/1  "TOF_Data"
  TD_baro/1(vH_TOF_TD) -> Scope/1, Bus Creator1/1  "vH_TOF_m/s_TD"
  Gain/1 -> Sum/2, reinit_TOF/2(Data)  "TOF_Dist_m"
  Data Type Conversion/1 -> Bus Creator1/4  "TOF_sts"
  QGC_sensor_reinit/1 -> reinit_TOF/1(QGC_sensor_reinit)
  reinit_TOF/1(dataout) -> Scope1/1, Sum/1
  Sum/1 -> Scope1/2, Data Type Conversion1/1  "TOF_Dist_m"

== system VB_RI_EKF_GNSS_INS25/No.1_Sensor_Data_Process1/baro_Data_Process ==
  baro : Inport
  QGC_sensor_reinit : Inport  Port=2
  baro_tem : Inport  Port=3
  Bus Creator : BusCreator  Inputs=2
  Constant : Constant  Value=0  OutDataTypeStr=single
  From Workspace : FromWorkspace  Commented=on  VariableName=[All.t',All.Alt_Ps]
  Gain : Gain  Gain=0.01
  Pressure2Height : Subsystem
  Scope : Scope
  Scope1 : Scope  Commented=on  NumInputPorts=2
  Sum : Sum  Inputs=|+-
  Sum1 : Sum  Commented=on  Inputs=|+-
  Sum2 : Sum  Inputs=|+-
  Switch : Switch  Criteria=u2 > Threshold  Threshold=31  SaturateOnIntegerOverflow=off  InputSameDT=off
  TD_baro : Subsystem
  TemCompensate1 : Subsystem
  reinit_baro0 : Subsystem
  reinit_baro1 : Subsystem  Commented=on
  BARO_Data : Outport  PortDimensions=2
  wires:
  Sum1/1 -> Scope1/1
  reinit_baro1/1(dataout) -> Sum1/2
  From Workspace/1 -> Sum1/1, reinit_baro1/2(Data)
  TD_baro/1(vH_baro_TD) -> Bus Creator/1  "vH_baro_m/s_TD"
  Gain/1 -> Pressure2Height/1(baro)
  Bus Creator/1 -> BARO_Data/1
  QGC_sensor_reinit/1 -> reinit_baro0/1(QGC_sensor_reinit), reinit_baro1/1(QGC_sensor_reinit)
  reinit_baro0/1(dataout) -> Sum/2
  Sum/1 -> Bus Creator/2, Scope/1, Scope1/2  "H_baro_TD"
  TD_baro/2(H_baro_TD) -> Sum2/1  "H_baro_TD"
  Sum2/1 -> reinit_baro0/2(Data), Sum/1
  TemCompensate1/1(bias) -> Switch/3
  Constant/1 -> Switch/1
  baro/1 -> Gain/1  "AFC4"
  Switch/1 -> Sum2/2
  Pressure2Height/1(H_baro) -> TD_baro/1(H_baro)  "AFC4"
  baro_tem/1 -> Switch/2, TemCompensate1/1(baro_tem)  "AFCbarotem"

== system VB_RI_EKF_GNSS_INS25/No.1_Sensor_Data_Process2/GPS_Data_Process ==
  note: GPS_fixtype:
      | 0: 定位不可用或无效
      | 1:单点定位
      | 2:伪距差分
      | 4:RTK固定解
  GPS_Vecef_m/s : Inport
  GPS_LLA_rad : Inport  Port=2
  GPS_fixtype : Inport  Port=3
  hdop_GPS : Inport  Port=4
  QGC_sensor_reinit : Inport  Port=5
  GPS0 : Inport  Port=6
  Bus Creator : BusCreator  Inputs=13
  Demux : Demux  Outputs=3
  Demux1 : Demux  Outputs=3
  Demux3 : Demux  Outputs=3
  GPS_fixtype1 : InportShadow  Port=3
  LLA2NED : Subsystem
  heading_GPS : Subsystem
  GPS_Data : Outport
  wires:
  hdop_GPS/1 -> Bus Creator/13  "hdop_GPS"
  heading_GPS/2(heading_GPS_valid) -> Bus Creator/11  "heading_GPS_valid"
  heading_GPS/1(heading_GPS_rad) -> Bus Creator/10  "heading_GPS_rad"
  LLA2NED/2(gpsvNEDout) -> heading_GPS/1(Vned), Demux/1
  GPS_Vecef_m/s/1 -> LLA2NED/3(GPS_Vecef_m/s)
  Demux1/3 -> Bus Creator/6  "pos_D_gps"
  Demux1/2 -> Bus Creator/5  "pos_E_gps"
  Demux1/1 -> Bus Creator/4  "pos_N_gps"
  QGC_sensor_reinit/1 -> LLA2NED/4(QGC_sensor_reinit)  "QGC_sensor_reinit"
  GPS_fixtype/1 -> Bus Creator/12  "fixtype_gps"
  Demux3/1 -> Bus Creator/1  "lat_gps"
  Demux3/2 -> Bus Creator/2  "lon_gps"
  Demux/2 -> Bus Creator/8  "ve_gps"
  GPS_LLA_rad/1 -> LLA2NED/1(gps_LLA_rad), Demux3/1
  Demux/1 -> Bus Creator/7  "vn_gps"
  Demux/3 -> Bus Creator/9  "vd_gps"
  Demux3/3 -> Bus Creator/3  "H_gps"
  Bus Creator/1 -> GPS_Data/1
  GPS_fixtype1/1 -> LLA2NED/2(GPSfixtype)  "fixtype_gps"
  LLA2NED/1("gpsposNEDout ") -> Demux1/1
  GPS0/1 -> LLA2NED/5(GPS0)

== system VB_RI_EKF_GNSS_INS25/No.1_Sensor_Data_Process2/IMU_Data_Process ==
  gyro_B_rad/s_ori : Inport
  accl_B_m/s_ori : Inport  Port=2
  Bias Eliminate : Subsystem
  Bus Creator : BusCreator  Inputs=2
  accl_preprocessing2 : Subsystem  Commented=on
  gyro_preprocessing2 : Subsystem  Commented=on
  IMU_Data : Outport  PortDimensions=6
  wires:
  gyro_B_rad/s_ori/1 -> Bias Eliminate/1(gyro_B_rad/s_ori)  "gyro_B_rad/s_LPF"
  Bias Eliminate/1(Out1) -> Bus Creator/1  "gyro_B_rad/s_LPF"
  accl_B_m/s_ori/1 -> Bus Creator/2  "accl_B_m/s2_LPF"
  Bus Creator/1 -> IMU_Data/1

== system VB_RI_EKF_GNSS_INS25/No.1_Sensor_Data_Process2/Magn_Data_Process ==
  magn_B_guass_ori : Inport
  Data Type Conversion : DataTypeConversion  OutDataTypeStr=single  SaturateOnIntegerOverflow=off  RndMeth=Floor
  MATLAB Function1 : MATLAB Function  Commented=on  TreatAsAtomicUnit=on
  Magn_preprocessing : Subsystem
  MAGN_Data : Outport
  wires:
  magn_B_guass_ori/1 -> Data Type Conversion/1, Magn_preprocessing/1(Magn_B_rad/s_ori)
  Data Type Conversion/1 -> MAGN_Data/1

== system VB_RI_EKF_GNSS_INS25/No.1_Sensor_Data_Process2/Subsystem ==
  Vairspeed : Inport
  Constant : Constant  Value=0  OutDataTypeStr=single
  Mux : Mux  Inputs=3
  TD_baro : Subsystem
  Terminator : Terminator
  VairspeedData : Outport
  wires:
  TD_baro/2(H_baro_TD) -> Mux/1
  Constant/1 -> Mux/3, Mux/2
  Mux/1 -> VairspeedData/1  "VairspeedData"
  Vairspeed/1 -> TD_baro/1(H_baro)
  TD_baro/1(vH_baro_TD) -> Terminator/1  "vH_baro_m/s_TD"

== system VB_RI_EKF_GNSS_INS25/No.1_Sensor_Data_Process2/TOF_Data_Process ==
  TOF_mm_ori : Inport
  QGC_sensor_reinit : Inport  Port=2
  Bus Creator1 : BusCreator  Inputs=4
  Data Type Conversion : DataTypeConversion  OutDataTypeStr=uint8  SaturateOnIntegerOverflow=off  RndMeth=Floor
  Data Type Conversion1 : DataTypeConversion  OutDataTypeStr=single  SaturateOnIntegerOverflow=off  RndMeth=Floor
  Demux : Demux  Outputs=3
  Gain : Gain  Gain=0.01
  Scope : Scope  NumInputPorts=2
  Scope1 : Scope  NumInputPorts=2
  Sum : Sum  Inputs=|-+
  TD_baro : Subsystem
  reinit_TOF : Subsystem
  TOF_Data : Outport
  wires:
  Sum/1 -> Data Type Conversion1/1, Scope1/2  "TOF_Dist_m"
  reinit_TOF/1(dataout) -> Sum/1, Scope1/1
  QGC_sensor_reinit/1 -> reinit_TOF/1(QGC_sensor_reinit)
  Data Type Conversion/1 -> Bus Creator1/4  "TOF_sts"
  Gain/1 -> reinit_TOF/2(Data), Sum/2  "TOF_Dist_m"
  TD_baro/1(vH_TOF_TD) -> Bus Creator1/1, Scope/1  "vH_TOF_m/s_TD"
  Bus Creator1/1 -> TOF_Data/1  "TOF_Data"
  Demux/2 -> Bus Creator1/3  "TOF_Inten"
  TOF_mm_ori/1 -> Demux/1
  Demux/1 -> Gain/1
  Demux/3 -> Data Type Conversion/1  "TOF_sts"
  TD_baro/2(H_TOF_TD) -> Scope/2, Bus Creator1/2  "H_TOF_TD"
  Data Type Conversion1/1 -> TD_baro/1(H_TOF)  "补偿姿态前"

== system VB_RI_EKF_GNSS_INS25/No.1_Sensor_Data_Process2/baro_Data_Process ==
  baro : Inport
  QGC_sensor_reinit : Inport  Port=2
  baro_tem : Inport  Port=3
  Bus Creator : BusCreator  Inputs=2
  Constant : Constant  Value=0  OutDataTypeStr=single
  From Workspace : FromWorkspace  Commented=on  VariableName=[All.t',All.Alt_Ps]
  Gain : Gain  Gain=0.01
  Pressure2Height : Subsystem
  Scope : Scope
  Scope1 : Scope  Commented=on  NumInputPorts=2
  Sum : Sum  Inputs=|+-
  Sum1 : Sum  Commented=on  Inputs=|+-
  Sum2 : Sum  Inputs=|+-
  Switch : Switch  Criteria=u2 > Threshold  Threshold=31  SaturateOnIntegerOverflow=off  InputSameDT=off
  TD_baro : Subsystem
  TemCompensate1 : Subsystem
  reinit_baro0 : Subsystem
  reinit_baro1 : Subsystem  Commented=on
  BARO_Data : Outport  PortDimensions=2
  wires:
  baro_tem/1 -> TemCompensate1/1(baro_tem), Switch/2  "AFCbarotem"
  Pressure2Height/1(H_baro) -> TD_baro/1(H_baro)  "AFC4"
  Switch/1 -> Sum2/2
  baro/1 -> Gain/1  "AFC4"
  Constant/1 -> Switch/1
  TemCompensate1/1(bias) -> Switch/3
  Sum2/1 -> Sum/1, reinit_baro0/2(Data)
  TD_baro/2(H_baro_TD) -> Sum2/1  "H_baro_TD"
  Sum/1 -> Scope1/2, Scope/1, Bus Creator/2  "H_baro_TD"
  reinit_baro0/1(dataout) -> Sum/2
  QGC_sensor_reinit/1 -> reinit_baro1/1(QGC_sensor_reinit), reinit_baro0/1(QGC_sensor_reinit)
  Bus Creator/1 -> BARO_Data/1
  Gain/1 -> Pressure2Height/1(baro)
  TD_baro/1(vH_baro_TD) -> Bus Creator/1  "vH_baro_m/s_TD"
  From Workspace/1 -> reinit_baro1/2(Data), Sum1/1
  reinit_baro1/1(dataout) -> Sum1/2
  Sum1/1 -> Scope1/1

== system VB_RI_EKF_GNSS_INS25/No.1_Sensor_Data_Process4/GPS_Data_Process ==
  note: GPS_fixtype:
      | 0: 定位不可用或无效
      | 1:单点定位
      | 2:伪距差分
      | 4:RTK固定解
  GPS_Vecef_m/s : Inport
  GPS_LLA_rad : Inport  Port=2
  GPS_fixtype : Inport  Port=3
  hdop_GPS : Inport  Port=4
  QGC_sensor_reinit : Inport  Port=5
  Bus Creator : BusCreator  Inputs=13
  Demux : Demux  Outputs=3
  Demux1 : Demux  Outputs=3
  Demux3 : Demux  Outputs=3
  GPS_fixtype1 : InportShadow  Port=3
  LLA2NED : Subsystem
  heading_GPS : Subsystem
  GPS_Data : Outport
  GPS0 : Outport  Port=2
  GPS_noerr : Outport  Port=3
  wires:
  LLA2NED/4(gpsposNED_noerr) -> GPS_noerr/1
  LLA2NED/3(GPS0) -> GPS0/1
  LLA2NED/1("gpsposNEDout ") -> Demux1/1
  GPS_fixtype1/1 -> LLA2NED/2(GPSfixtype)  "fixtype_gps"
  Bus Creator/1 -> GPS_Data/1
  Demux3/3 -> Bus Creator/3  "H_gps"
  Demux/3 -> Bus Creator/9  "vd_gps"
  Demux/1 -> Bus Creator/7  "vn_gps"
  GPS_LLA_rad/1 -> Demux3/1, LLA2NED/1(gps_LLA_rad)
  Demux/2 -> Bus Creator/8  "ve_gps"
  Demux3/2 -> Bus Creator/2  "lon_gps"
  Demux3/1 -> Bus Creator/1  "lat_gps"
  GPS_fixtype/1 -> Bus Creator/12  "fixtype_gps"
  QGC_sensor_reinit/1 -> LLA2NED/4(QGC_sensor_reinit)  "QGC_sensor_reinit"
  Demux1/1 -> Bus Creator/4  "pos_N_gps"
  Demux1/2 -> Bus Creator/5  "pos_E_gps"
  Demux1/3 -> Bus Creator/6  "pos_D_gps"
  GPS_Vecef_m/s/1 -> LLA2NED/3(GPS_Vecef_m/s)
  LLA2NED/2(gpsvNEDout) -> Demux/1, heading_GPS/1(Vned)
  heading_GPS/1(heading_GPS_rad) -> Bus Creator/10  "heading_GPS_rad"
  heading_GPS/2(heading_GPS_valid) -> Bus Creator/11  "heading_GPS_valid"
  hdop_GPS/1 -> Bus Creator/13  "hdop_GPS"

== system VB_RI_EKF_GNSS_INS25/No.1_Sensor_Data_Process4/IMU_Data_Process ==
  gyro_B_rad/s_ori : Inport
  accl_B_m/s_ori : Inport  Port=2
  Bias Eliminate : Subsystem
  Bus Creator : BusCreator  Inputs=2
  accl_preprocessing2 : Subsystem  Commented=on
  gyro_preprocessing2 : Subsystem  Commented=on
  IMU_Data : Outport  PortDimensions=6
  wires:
  Bus Creator/1 -> IMU_Data/1
  accl_B_m/s_ori/1 -> Bus Creator/2  "accl_B_m/s2_LPF"
  Bias Eliminate/1(Out1) -> Bus Creator/1  "gyro_B_rad/s_LPF"
  gyro_B_rad/s_ori/1 -> Bias Eliminate/1(gyro_B_rad/s_ori)  "gyro_B_rad/s_LPF"

== system VB_RI_EKF_GNSS_INS25/No.1_Sensor_Data_Process4/Magn_Data_Process ==
  magn_B_guass_ori : Inport
  Data Type Conversion : DataTypeConversion  OutDataTypeStr=single  SaturateOnIntegerOverflow=off  RndMeth=Floor
  MATLAB Function1 : MATLAB Function  Commented=on  TreatAsAtomicUnit=on
  Magn_preprocessing : Subsystem
  MAGN_Data : Outport
  wires:
  Data Type Conversion/1 -> MAGN_Data/1
  magn_B_guass_ori/1 -> Magn_preprocessing/1(Magn_B_rad/s_ori), Data Type Conversion/1

== system VB_RI_EKF_GNSS_INS25/No.1_Sensor_Data_Process4/Subsystem ==
  Vairspeed : Inport
  Constant : Constant  Value=0  OutDataTypeStr=single
  Mux : Mux  Inputs=3
  TD_baro : Subsystem
  Terminator : Terminator
  VairspeedData : Outport
  wires:
  TD_baro/1(vH_baro_TD) -> Terminator/1  "vH_baro_m/s_TD"
  Vairspeed/1 -> TD_baro/1(H_baro)
  Mux/1 -> VairspeedData/1  "VairspeedData"
  Constant/1 -> Mux/2, Mux/3
  TD_baro/2(H_baro_TD) -> Mux/1

== system VB_RI_EKF_GNSS_INS25/No.1_Sensor_Data_Process4/TOF_Data_Process ==
  TOF_mm_ori : Inport
  QGC_sensor_reinit : Inport  Port=2
  Bus Creator1 : BusCreator  Inputs=4
  Data Type Conversion : DataTypeConversion  OutDataTypeStr=uint8  SaturateOnIntegerOverflow=off  RndMeth=Floor
  Data Type Conversion1 : DataTypeConversion  OutDataTypeStr=single  SaturateOnIntegerOverflow=off  RndMeth=Floor
  Demux : Demux  Outputs=3
  Gain : Gain  Gain=0.01
  Scope : Scope  NumInputPorts=2
  Scope1 : Scope  NumInputPorts=2
  Sum : Sum  Inputs=|-+
  TD_baro : Subsystem
  reinit_TOF : Subsystem
  TOF_Data : Outport
  wires:
  Data Type Conversion1/1 -> TD_baro/1(H_TOF)  "补偿姿态前"
  TD_baro/2(H_TOF_TD) -> Bus Creator1/2, Scope/2  "H_TOF_TD"
  Demux/3 -> Data Type Conversion/1  "TOF_sts"
  Demux/1 -> Gain/1
  TOF_mm_ori/1 -> Demux/1
  Demux/2 -> Bus Creator1/3  "TOF_Inten"
  Bus Creator1/1 -> TOF_Data/1  "TOF_Data"
  TD_baro/1(vH_TOF_TD) -> Scope/1, Bus Creator1/1  "vH_TOF_m/s_TD"
  Gain/1 -> Sum/2, reinit_TOF/2(Data)  "TOF_Dist_m"
  Data Type Conversion/1 -> Bus Creator1/4  "TOF_sts"
  QGC_sensor_reinit/1 -> reinit_TOF/1(QGC_sensor_reinit)
  reinit_TOF/1(dataout) -> Scope1/1, Sum/1
  Sum/1 -> Scope1/2, Data Type Conversion1/1  "TOF_Dist_m"

== system VB_RI_EKF_GNSS_INS25/No.1_Sensor_Data_Process4/baro_Data_Process ==
  baro : Inport
  QGC_sensor_reinit : Inport  Port=2
  baro_tem : Inport  Port=3
  Bus Creator : BusCreator  Inputs=2
  Constant : Constant  Value=0  OutDataTypeStr=single
  From Workspace : FromWorkspace  Commented=on  VariableName=[All.t',All.Alt_Ps]
  Gain : Gain  Gain=0.01
  Pressure2Height : Subsystem
  Scope : Scope
  Scope1 : Scope  Commented=on  NumInputPorts=2
  Sum : Sum  Inputs=|+-
  Sum1 : Sum  Commented=on  Inputs=|+-
  Sum2 : Sum  Inputs=|+-
  Switch : Switch  Criteria=u2 > Threshold  Threshold=31  SaturateOnIntegerOverflow=off  InputSameDT=off
  TD_baro : Subsystem
  TemCompensate1 : Subsystem
  reinit_baro0 : Subsystem
  reinit_baro1 : Subsystem  Commented=on
  BARO_Data : Outport  PortDimensions=2
  wires:
  Sum1/1 -> Scope1/1
  reinit_baro1/1(dataout) -> Sum1/2
  From Workspace/1 -> Sum1/1, reinit_baro1/2(Data)
  TD_baro/1(vH_baro_TD) -> Bus Creator/1  "vH_baro_m/s_TD"
  Gain/1 -> Pressure2Height/1(baro)
  Bus Creator/1 -> BARO_Data/1
  QGC_sensor_reinit/1 -> reinit_baro0/1(QGC_sensor_reinit), reinit_baro1/1(QGC_sensor_reinit)
  reinit_baro0/1(dataout) -> Sum/2
  Sum/1 -> Bus Creator/2, Scope/1, Scope1/2  "H_baro_TD"
  TD_baro/2(H_baro_TD) -> Sum2/1  "H_baro_TD"
  Sum2/1 -> reinit_baro0/2(Data), Sum/1
  TemCompensate1/1(bias) -> Switch/3
  Constant/1 -> Switch/1
  baro/1 -> Gain/1  "AFC4"
  Switch/1 -> Sum2/2
  Pressure2Height/1(H_baro) -> TD_baro/1(H_baro)  "AFC4"
  baro_tem/1 -> Switch/2, TemCompensate1/1(baro_tem)  "AFCbarotem"

== system VB_RI_EKF_GNSS_INS25/RI EKF_AOA_LSTM/Bus_Constructor ==
  INSstate : Inport
  Bus Creator : BusCreator  Inputs=1
  Bus Creator1 : BusCreator  Inputs=3
  Bus Creator2 : BusCreator  Inputs=6
  Bus Creator3 : BusCreator  Inputs=3
  Bus Creator4 : BusCreator  Inputs=1
  Bus Selector : BusSelector  OutputSignals=RotationData.DCM_b_n,INSstate_v,INSstste_p,INSstate_dg,INSstate_da,INSstate_dm,INSstate_Rab,vel_wind_NED
  Data Store Read : DataStoreRead  DataStoreName=GPS_enable_RIEKF  IndexOptions=Index vector (dialog)  Indices=1  OutputSizes=1
  Demux : Demux  Outputs=3
  Demux1 : Demux  Outputs=3
  Demux2 : Demux  Outputs=3
  Direction Cosine Matrix to Rotation Angles : sharedtransform/Direction Cosine Matrix to Rotation Angles  rotationOrder=ZYX  aMode=aMode  action=None  tolerance=eps(2)
      settings: LibrarySourceBlock=|
      | aerolibtransform2/Direction Cosine Matrix
      | to Rotation Angles
  Gain : Gain  Gain=-1
  Radians to Degrees1 : simulink_extras/Transformations/Radians to Degrees
  Scope : Scope
  Terminator : Terminator
  Transpose1 : Math  Operator=transpose
  TranslationData : Outport
  RotationData : Outport  Port=2
  INSbiasData : Outport  Port=3
  AOA/SA/Wind : Outport  Port=4
  GNSS enable flag : Outport  Port=5
  wires:
  Bus Selector/5 -> Bus Creator1/2  "<INSstate_da>"
  Bus Selector/4 -> Bus Creator1/1  "<INSstate_dg>"
  Bus Selector/3 -> Demux1/1  "<INSstste_p>"
  Bus Creator/1 -> RotationData/1
  Bus Selector/1 -> Bus Creator/1  "<DCM_b_n>"
  INSstate/1 -> Bus Selector/1
  Demux/2 -> Bus Creator2/2  "ve_m/s"
  Bus Creator2/1 -> TranslationData/1
  Demux/3 -> Bus Creator2/3  "vd_m/s"
  Demux1/2 -> Bus Creator2/5  "pe_m"
  Demux1/1 -> Bus Creator2/4  "pn_m"
  Demux1/3 -> Bus Creator2/6  "pd_m"
  Bus Selector/2 -> Demux/1  "<INSstate_v>"
  Demux/1 -> Bus Creator2/1  "vn_m/s"
  Bus Selector/6 -> Bus Creator1/3  "<INSstate_dm>"
  Bus Creator1/1 -> INSbiasData/1
  Bus Selector/7 -> Transpose1/1  "<INSstate_Rab>"
  Bus Selector/8 -> Scope/1, Bus Creator3/3  "<vel_wind_NED>"
  Direction Cosine Matrix to Rotation Angles/1 -> Radians to Degrees1/1
  Transpose1/1 -> Direction Cosine Matrix to Rotation Angles/1
  Radians to Degrees1/1 -> Demux2/1
  Demux2/2 -> Gain/1
  Demux2/3 -> Terminator/1
  Demux2/1 -> Bus Creator3/2  "SA"
  Gain/1 -> Bus Creator3/1  "AOA"
  Bus Creator3/1 -> AOA/SA/Wind/1
  Data Store Read/1 -> Bus Creator4/1  "GNSS enable flag"
  Bus Creator4/1 -> GNSS enable flag/1
